simulink model "Checkpoint2"  (R2024a)
settings: Solver=VariableStepAuto  StartTime=0.0  StopTime=10.0  MaxStep=1e-3  RelTol=1e-3
PreLoadFcn:
  | load('PROP_DATA_INTRO')
undefined symbols (not defined in the file): PropData
libraries: simulink x1

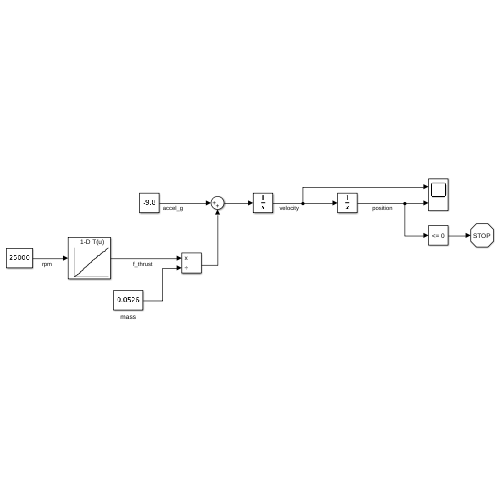
[thumbnail: Simulink's stored preview of the top-level diagram]
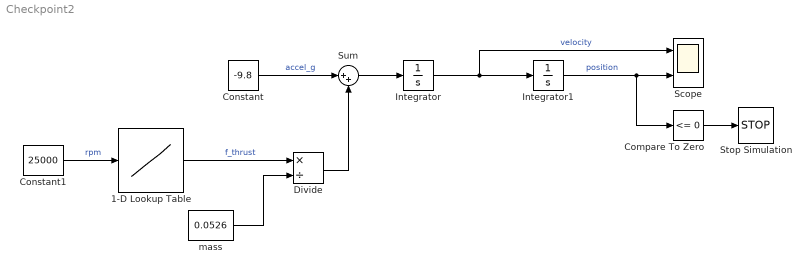
== system Checkpoint2 ==
  1-D Lookup Table : Lookup_n-D  NumberOfTableDimensions=1  BreakpointsForDimension1=PropData.rpm  Table=PropData.liftForce_N  InternalRulePriority=Speed  RndMeth=Simplest
  Compare To Zero : simulink/Logic and Bit Operations/Compare To Zero  relop=<=  OutDataTypeStr=boolean
  Constant : Constant  Value=-9.8
  Constant1 : Constant  Value=25000
  Divide : Product  Inputs=*/
  Integrator : Integrator  InitialCondition=0.5
  Integrator1 : Integrator  InitialCondition=1
  Scope : Scope  NumInputPorts=2
  Stop Simulation : Stop
  Sum : Sum  Inputs=|++
  mass : Constant  Value=0.0526
  wires:
  Integrator/1 -> Scope/1, Integrator1/1  "velocity"
  Integrator1/1 -> Compare To Zero/1, Scope/2  "position"
  Compare To Zero/1 -> Stop Simulation/1
  Sum/1 -> Integrator/1
  Constant/1 -> Sum/1  "accel_g"
  Constant1/1 -> 1-D Lookup Table/1  "rpm"
  1-D Lookup Table/1 -> Divide/1  "f_thrust"
  Divide/1 -> Sum/2
  mass/1 -> Divide/2
